simulink subsystem "bit64_binary_index_search"  (R2021b)
settings: Solver=VariableStepAuto  StartTime=0.0  StopTime=10.0  RelTol=1e-3
libraries: hdlsllib x1
settings Model: Creator=torha  LastModifiedBy=torha
settings SolverCC: AlgebraicLoopSolver=TrustRegion
settings DebuggingCC: SFMachineParentedDataDiag=warning

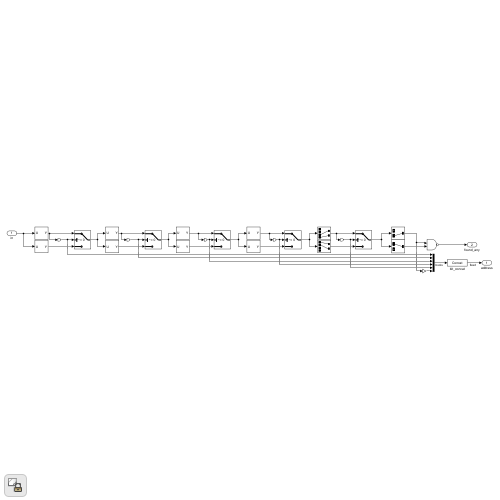
[thumbnail: Simulink's stored preview of the top-level diagram]
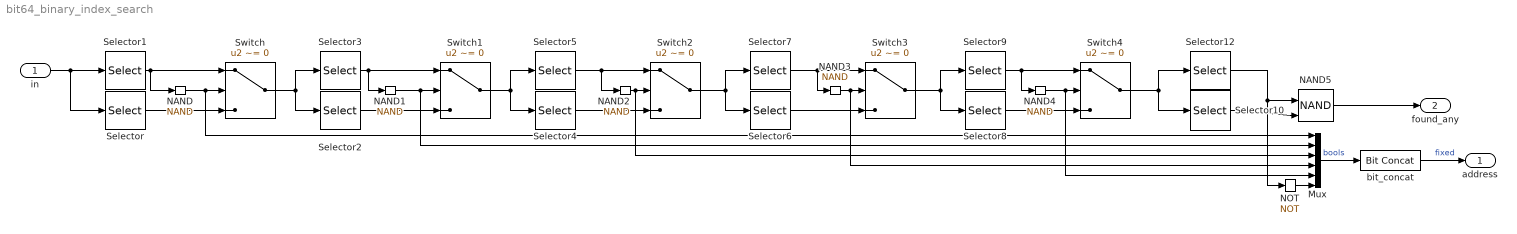
== system bit64_binary_index_search ==
  in : Inport
  Mux : Mux  Inputs=6
  NAND{,1..4} (5 alike) : Logic  Operator=NAND  Inputs=1  IconShape=distinctive  AllPortsSameDT=off  OutDataTypeStr=boolean
  NAND5 : Logic  Operator=NAND  IconShape=distinctive  AllPortsSameDT=off  OutDataTypeStr=boolean
  NOT : Logic  Operator=NOT  IconShape=distinctive  AllPortsSameDT=off  OutDataTypeStr=boolean
  Selector : Selector  IndexOptions=Starting index (dialog)  Indices=1  OutputSizes=32
  Selector1 : Selector  IndexOptions=Starting index (dialog)  Indices=33  OutputSizes=32
  Selector10 : Selector  InputPortWidth=2  IndexOptions=Index vector (dialog)  Indices=1  OutputSizes=1
  Selector12 : Selector  InputPortWidth=2  IndexOptions=Index vector (dialog)  Indices=2  OutputSizes=1
  Selector2 : Selector  IndexOptions=Starting index (dialog)  Indices=1  OutputSizes=16
  Selector3 : Selector  IndexOptions=Starting index (dialog)  Indices=17  OutputSizes=16
  Selector4 : Selector  IndexOptions=Starting index (dialog)  Indices=1  OutputSizes=8
  Selector5 : Selector  IndexOptions=Starting index (dialog)  Indices=9  OutputSizes=8
  Selector6 : Selector  InputPortWidth=8  IndexOptions=Starting index (dialog)  Indices=1  OutputSizes=4
  Selector7 : Selector  InputPortWidth=8  IndexOptions=Starting index (dialog)  Indices=5  OutputSizes=4
  Selector8 : Selector  InputPortWidth=4  IndexOptions=Starting index (dialog)  Indices=1  OutputSizes=2
  Selector9 : Selector  InputPortWidth=4  IndexOptions=Starting index (dialog)  Indices=3  OutputSizes=2
  Switch : Switch  Criteria=u2 ~= 0  Threshold=1
  Switch{1..4} (4 alike) : Switch  Criteria=u2 ~= 0
  bit_concat : hdlsllib/Logic and Bit Operations/Bit Concat  numInputs=1
  address : Outport
  found_any : Outport  Port=2
  wires:
  Mux/1 -> bit_concat/1  "bools"
  NAND5/1 -> found_any/1
  Switch4/1 -> Selector10/1, Selector12/1
  NAND4/1 -> Switch4/2, Mux/5
  Selector8/1 -> Switch4/3
  Switch3/1 -> Selector9/1, Selector8/1
  Switch2/1 -> Selector7/1, Selector6/1
  Selector6/1 -> Switch3/3
  NAND3/1 -> Switch3/2, Mux/4
  Switch1/1 -> Selector5/1, Selector4/1
  Selector4/1 -> Switch2/3
  NAND2/1 -> Switch2/2, Mux/3
  NAND1/1 -> Switch1/2, Mux/2
  Switch/1 -> Selector3/1, Selector2/1
  Selector3/1 -> NAND1/1, Switch1/1
  Selector2/1 -> Switch1/3
  Selector1/1 -> Switch/1, NAND/1
  Selector/1 -> Switch/3
  bit_concat/1 -> address/1  "fixed"
  in/1 -> Selector1/1, Selector/1
  Selector5/1 -> Switch2/1, NAND2/1
  Selector7/1 -> Switch3/1, NAND3/1
  Selector9/1 -> Switch4/1, NAND4/1
  NAND/1 -> Switch/2, Mux/1
  Selector12/1 -> NAND5/1, NOT/1
  Selector10/1 -> NAND5/2
  NOT/1 -> Mux/6
